simulink model "example03"  (R2022a)
settings: Solver=VariableStepAuto  StartTime=0.0  StopTime=10.0  RelTol=1e-3
settings Model: Creator=mluser  LastModifiedBy=cunis
settings ModelReferenceCC: EnableRefExpFcnMdlSchedulingChecks=off
settings RTWCC: Description=Generic Real-Time Target

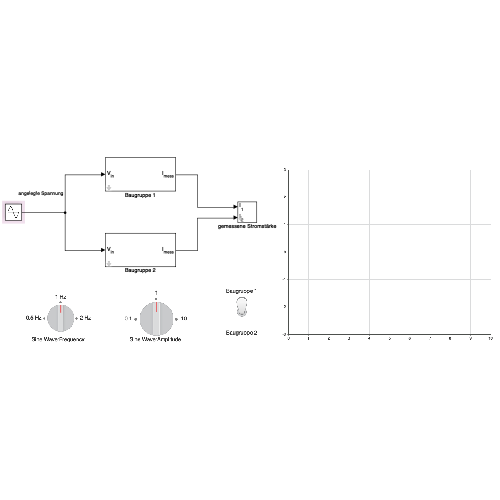
[thumbnail: Simulink's stored preview of the top-level diagram]
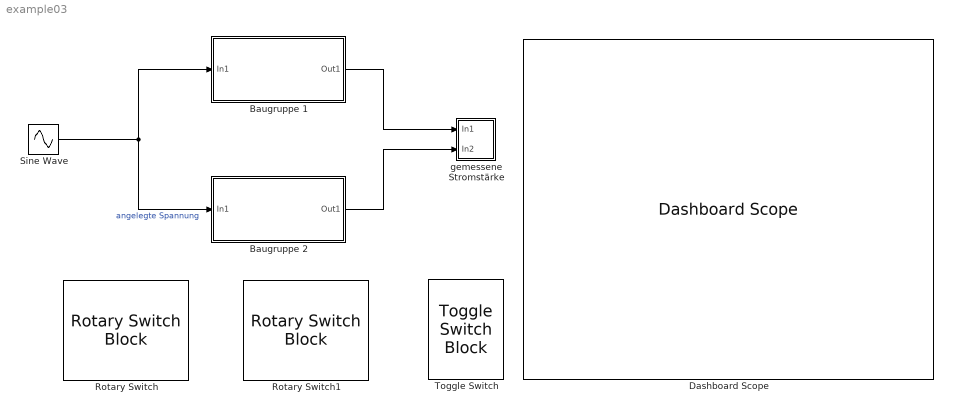
== system example03 ==
  Baugruppe 1 : Subsystem
      mask Display:
      | port_label('input', 1, 'V_{in}', 'interpreter', 'tex');
      | port_label('output', 1, 'I_{mess}', 'interpreter', 'tex');
  Baugruppe 2 : Subsystem
      mask Display:
      | port_label('input', 1, 'V_{in}', 'interpreter', 'tex');
      | port_label('output', 1, 'I_{mess}', 'interpreter', 'tex');
  Dashboard Scope : DashboardScope
  Rotary Switch : RotarySwitchBlock  LabelPosition=Bottom
      settings: Values={{'0.5 Hz', '1 Hz', '2 Hz'}, [0.5 1 2]}
  Rotary Switch1 : RotarySwitchBlock  LabelPosition=Bottom
      settings: Values={{'0.1', '1', '10'}, [0.1 1 10]}
  Sine Wave : Sin  SampleTime=0
  Toggle Switch : ToggleSwitchBlock  LabelPosition=Hide
      settings: Values={{'Baugruppe 2', 'Baugruppe 1'}, [0 1]}
  gemessene Stromstärke : Subsystem
      mask Display:
      | port_label('input', 1, 'I_1', 'interpreter', 'tex');
      | port_label('input', 2, 'I_2', 'interpreter', 'tex');
  wires:
  Sine Wave/1 -> Baugruppe 2/1(In1), Baugruppe 1/1(In1)  "angelegte Spannung"
  Baugruppe 1/1(Out1) -> gemessene Stromstärke/1(In1)
  Baugruppe 2/1(Out1) -> gemessene Stromstärke/2(In2)

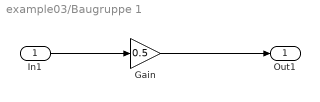
== system example03/Baugruppe 1 ==
  In1 : Inport
  Gain : Gain  Gain=0.5
  Out1 : Outport
  wires:
  In1/1 -> Gain/1
  Gain/1 -> Out1/1

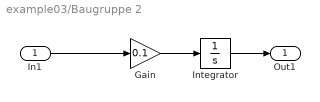
== system example03/Baugruppe 2 ==
  In1 : Inport
  Gain : Gain  Gain=0.1
  Integrator : Integrator
  Out1 : Outport
  wires:
  In1/1 -> Gain/1
  Gain/1 -> Integrator/1
  Integrator/1 -> Out1/1

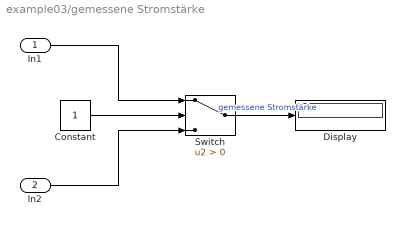
== system example03/gemessene Stromstärke ==
  In1 : Inport
  In2 : Inport  Port=2
  Constant : Constant
  Display : Display
  Switch : Switch  Criteria=u2 > Threshold  SaturateOnIntegerOverflow=off  InputSameDT=off
  wires:
  In1/1 -> Switch/1
  In2/1 -> Switch/3
  Switch/1 -> Display/1  "gemessene Stromstärke"
  Constant/1 -> Switch/2
